simulink model "test_mdl_NI"  (R2018a)
settings: Solver=VariableStepAuto  StartTime=0.0  StopTime=10.0  RelTol=1e-3
(part 7 of 24)

== system test_mdl_NI/Subsystem/ABS_ESC/BrakeSysFeatures_2_Ox416 ==
  in_port : Inport
  Abs_B_Falt : Terminator
  BpedMove_D_Actl : Terminator
  BpedMove_No_Cnt : Terminator
  BrkBstrVac_B_Rq : Terminator
  BrkLamp_B_Rq : Terminator
  ChimeBrk_B_Rq : Terminator
  DrvAntiLckLamp_D_Rq : Terminator
  DrvHdcLampInfo_D_Rq : Terminator
  DrvHdcMsg_D_Rq : Terminator
  DrvHdcWarnInfo_D_Rq : Terminator
  DrvSlipCtlLamp_D_Rq : Terminator
  DrvSlipCtlMde_D_Ind : Terminator
  HILL_DESC_MC : Terminator
  HdcMde_D_Actl : Terminator
  HsaMde_D_Mem : Terminator
  RearDiffElckrOpen_B_Rq : Terminator
  RearDiffLck_Tq2_RqMx : Terminator
  StabCtlBrk_B_Avail : Terminator
  TCMode : Terminator
  TRLR_SWAY_CONFIG_STAT : Terminator
  TRLR_SWAY_EVNT_IN_PROG : Terminator
  bus_selector : BusSelector  OutputSignals=Abs_B_Falt,BpedMove_D_Actl,BpedMove_No_Cnt,BrkBstrVac_B_Rq,BrkLamp_B_Rq,ChimeBrk_B_Rq,DrvAntiLckLamp_D_Rq,DrvHdcLampInfo_D_Rq,DrvHdcMsg_D_Rq,DrvHdcWarnInfo_D_Rq,DrvSlipCtlLamp_D_Rq,DrvSlipCtlMde_D_Ind,HILL_DESC_MC,HdcMde_D_Actl,HsaMde_D_Mem,RearDiffElckrOpen_B_Rq,RearDiffLck_Tq2_RqMx,StabCtlBrk_B_Avail,TCMode,TRLR_SWAY_CONFIG_STAT,TRLR_SWAY_EVNT_IN_PROG
  wires:
  in_port/1 -> bus_selector/1  "BrakeSysFeatures_2_Ox416"
  bus_selector/1 -> Abs_B_Falt/1  "<Abs_B_Falt>"
  bus_selector/2 -> BpedMove_D_Actl/1  "<BpedMove_D_Actl>"
  bus_selector/3 -> BpedMove_No_Cnt/1  "<BpedMove_No_Cnt>"
  bus_selector/4 -> BrkBstrVac_B_Rq/1  "<BrkBstrVac_B_Rq>"
  bus_selector/5 -> BrkLamp_B_Rq/1  "<BrkLamp_B_Rq>"
  bus_selector/6 -> ChimeBrk_B_Rq/1  "<ChimeBrk_B_Rq>"
  bus_selector/7 -> DrvAntiLckLamp_D_Rq/1  "<DrvAntiLckLamp_D_Rq>"
  bus_selector/8 -> DrvHdcLampInfo_D_Rq/1  "<DrvHdcLampInfo_D_Rq>"
  bus_selector/9 -> DrvHdcMsg_D_Rq/1  "<DrvHdcMsg_D_Rq>"
  bus_selector/10 -> DrvHdcWarnInfo_D_Rq/1  "<DrvHdcWarnInfo_D_Rq>"
  bus_selector/11 -> DrvSlipCtlLamp_D_Rq/1  "<DrvSlipCtlLamp_D_Rq>"
  bus_selector/12 -> DrvSlipCtlMde_D_Ind/1  "<DrvSlipCtlMde_D_Ind>"
  bus_selector/13 -> HILL_DESC_MC/1  "<HILL_DESC_MC>"
  bus_selector/14 -> HdcMde_D_Actl/1  "<HdcMde_D_Actl>"
  bus_selector/15 -> HsaMde_D_Mem/1  "<HsaMde_D_Mem>"
  bus_selector/16 -> RearDiffElckrOpen_B_Rq/1  "<RearDiffElckrOpen_B_Rq>"
  bus_selector/17 -> RearDiffLck_Tq2_RqMx/1  "<RearDiffLck_Tq2_RqMx>"
  bus_selector/18 -> StabCtlBrk_B_Avail/1  "<StabCtlBrk_B_Avail>"
  bus_selector/19 -> TCMode/1  "<TCMode>"
  bus_selector/20 -> TRLR_SWAY_CONFIG_STAT/1  "<TRLR_SWAY_CONFIG_STAT>"
  bus_selector/21 -> TRLR_SWAY_EVNT_IN_PROG/1  "<TRLR_SWAY_EVNT_IN_PROG>"

== system test_mdl_NI/Subsystem/ABS_ESC/BrakeSysFeatures_3_Ox41E ==
  in_port : Inport
  AirDamUp_B_RqBrk : Terminator
  ApaBrk_D_Stat : Terminator
  AutoHoldMde_D_Ind : Terminator
  AutoHoldMsgTxt_D_Rq : Terminator
  AutoHoldSwMde_B_Ind : Terminator
  BrkBstrVac_D_Stat : Terminator
  CtaBrk_D_Stat : Terminator
  DrvSlipCtlMdeMsg_D_Rq : Terminator
  DrvSlipCtlOffLamp_D_Rq : Terminator
  RbaBrk_D_Stat : Terminator
  SelDrvMdeAwd_D_Rq : Terminator
  SelDrvMdeChassis2_D_Rq : Terminator
  SelDrvMdeChassis_D_Rq : Terminator
  TrailCtlMsgTxt_D_Rq : Terminator
  TrailCtl_D_Stat : Terminator
  bus_selector : BusSelector  OutputSignals=AirDamUp_B_RqBrk,ApaBrk_D_Stat,AutoHoldMde_D_Ind,AutoHoldMsgTxt_D_Rq,AutoHoldSwMde_B_Ind,BrkBstrVac_D_Stat,CtaBrk_D_Stat,DrvSlipCtlMdeMsg_D_Rq,DrvSlipCtlOffLamp_D_Rq,RbaBrk_D_Stat,SelDrvMdeAwd_D_Rq,SelDrvMdeChassis2_D_Rq,SelDrvMdeChassis_D_Rq,TrailCtlMsgTxt_D_Rq,TrailCtl_D_Stat
  wires:
  in_port/1 -> bus_selector/1  "BrakeSysFeatures_3_Ox41E"
  bus_selector/1 -> AirDamUp_B_RqBrk/1  "<AirDamUp_B_RqBrk>"
  bus_selector/2 -> ApaBrk_D_Stat/1  "<ApaBrk_D_Stat>"
  bus_selector/3 -> AutoHoldMde_D_Ind/1  "<AutoHoldMde_D_Ind>"
  bus_selector/4 -> AutoHoldMsgTxt_D_Rq/1  "<AutoHoldMsgTxt_D_Rq>"
  bus_selector/5 -> AutoHoldSwMde_B_Ind/1  "<AutoHoldSwMde_B_Ind>"
  bus_selector/6 -> BrkBstrVac_D_Stat/1  "<BrkBstrVac_D_Stat>"
  bus_selector/7 -> CtaBrk_D_Stat/1  "<CtaBrk_D_Stat>"
  bus_selector/8 -> DrvSlipCtlMdeMsg_D_Rq/1  "<DrvSlipCtlMdeMsg_D_Rq>"
  bus_selector/9 -> DrvSlipCtlOffLamp_D_Rq/1  "<DrvSlipCtlOffLamp_D_Rq>"
  bus_selector/10 -> RbaBrk_D_Stat/1  "<RbaBrk_D_Stat>"
  bus_selector/11 -> SelDrvMdeAwd_D_Rq/1  "<SelDrvMdeAwd_D_Rq>"
  bus_selector/12 -> SelDrvMdeChassis2_D_Rq/1  "<SelDrvMdeChassis2_D_Rq>"
  bus_selector/13 -> SelDrvMdeChassis_D_Rq/1  "<SelDrvMdeChassis_D_Rq>"
  bus_selector/14 -> TrailCtlMsgTxt_D_Rq/1  "<TrailCtlMsgTxt_D_Rq>"
  bus_selector/15 -> TrailCtl_D_Stat/1  "<TrailCtl_D_Stat>"

== system test_mdl_NI/Subsystem/ABS_ESC/BrakeSysFeatures_Ox415 ==
  in_port : Inport
  BrkFluidLvl_D_Stat : Terminator
  LsmcBrkDecel_D_Stat : Terminator
  VehStab_D_Stat : Terminator
  VehVActlBrk_D_Qf : Terminator
  VehVActlBrk_No_Cnt : Terminator
  VehVActlBrk_No_Cs : Terminator
  VehYawLin_W_Rq : Terminator
  VehYawNonLin_W_Rq : Terminator
  Veh_V_ActlBrk : Terminator
  bus_selector : BusSelector  OutputSignals=BrkFluidLvl_D_Stat,LsmcBrkDecel_D_Stat,VehStab_D_Stat,VehVActlBrk_D_Qf,VehVActlBrk_No_Cnt,VehVActlBrk_No_Cs,VehYawLin_W_Rq,VehYawNonLin_W_Rq,Veh_V_ActlBrk
  wires:
  in_port/1 -> bus_selector/1  "BrakeSysFeatures_Ox415"
  bus_selector/1 -> BrkFluidLvl_D_Stat/1  "<BrkFluidLvl_D_Stat>"
  bus_selector/2 -> LsmcBrkDecel_D_Stat/1  "<LsmcBrkDecel_D_Stat>"
  bus_selector/3 -> VehStab_D_Stat/1  "<VehStab_D_Stat>"
  bus_selector/4 -> VehVActlBrk_D_Qf/1  "<VehVActlBrk_D_Qf>"
  bus_selector/5 -> VehVActlBrk_No_Cnt/1  "<VehVActlBrk_No_Cnt>"
  bus_selector/6 -> VehVActlBrk_No_Cs/1  "<VehVActlBrk_No_Cs>"
  bus_selector/7 -> VehYawLin_W_Rq/1  "<VehYawLin_W_Rq>"
  bus_selector/8 -> VehYawNonLin_W_Rq/1  "<VehYawNonLin_W_Rq>"
  bus_selector/9 -> Veh_V_ActlBrk/1  "<Veh_V_ActlBrk>"

== system test_mdl_NI/Subsystem/ABS_ESC/DesiredTorqBrk_2_Ox214 ==
  in_port : Inport
  PrplWhlTot_Tq_RqMn : Terminator
  PrplWhlTqRqMn_No_Cnt : Terminator
  PrplWhlTqRqMn_No_Cs : Terminator
  RgenBrkDynoMde_B_Actl : Terminator
  RgenTqFalt_B_Actl : Terminator
  bus_selector : BusSelector  OutputSignals=PrplWhlTot_Tq_RqMn,PrplWhlTqRqMn_No_Cnt,PrplWhlTqRqMn_No_Cs,RgenBrkDynoMde_B_Actl,RgenTqFalt_B_Actl
  wires:
  in_port/1 -> bus_selector/1  "DesiredTorqBrk_2_Ox214"
  bus_selector/1 -> PrplWhlTot_Tq_RqMn/1  "<PrplWhlTot_Tq_RqMn>"
  bus_selector/2 -> PrplWhlTqRqMn_No_Cnt/1  "<PrplWhlTqRqMn_No_Cnt>"
  bus_selector/3 -> PrplWhlTqRqMn_No_Cs/1  "<PrplWhlTqRqMn_No_Cs>"
  bus_selector/4 -> RgenBrkDynoMde_B_Actl/1  "<RgenBrkDynoMde_B_Actl>"
  bus_selector/5 -> RgenTqFalt_B_Actl/1  "<RgenTqFalt_B_Actl>"

== system test_mdl_NI/Subsystem/ABS_ESC/DesiredTorqBrk_Ox213 ==
  in_port : Inport
  AbsActv_B_Actl : Terminator
  AccBrkActv_B_Actl : Terminator
  AccBrkDeny_B_Actl : Terminator
  AccBrkDis_B_Actl : Terminator
  AccBrkPrchgActv_B_Actl : Terminator
  AccBrkTotTqMn_B_Actl : Terminator
  AccBrkWarm_B_Actl : Terminator
  AccDis_B_ActlEpb : Terminator
  AccStopActv_B_ActlBrk : Terminator
  CcDis_B_Cmd : Terminator
  CmbbBaSensInc_B_Actl : Terminator
  CmbbBrkDecel_B_Actl : Terminator
  CmbbBrkDis_B_Actl : Terminator
  CmbbBrkPrchg_B_Actl : Terminator
  CmbbDeny_B_ActlBrk : Terminator
  LscmbBrkPrchg_B_Actl : Terminator
  LscmbbBaSensInc_B_Actl : Terminator
  LscmbbBrkDecel_B_Actl : Terminator
  LscmbbBrkDis_B_Actl : Terminator
  LscmbbDeny_B_ActlBrk : Terminator
  LscmbbMntr_B_Err : Terminator
  PrkBrkMsgTxt_D_Rq : Terminator
  PrkBrkRedLamp_D_Rq : Terminator
  PrkBrkStatus : Terminator
  PrkBrkYwLamp_D_Rq : Terminator
  PrplDrgCtlActv_B_Actl : Terminator
  PrplWhlTot_Tq_RqMx : Terminator
  StabCtlBrkActv_B_Actl : Terminator
  TracCtlPtActv_B_Actl : Terminator
  VehLongOvrGnd_A_Est : Terminator
  VehStop_D_Stat : Terminator
  bus_selector : BusSelector  OutputSignals=AbsActv_B_Actl,AccBrkActv_B_Actl,AccBrkDeny_B_Actl,AccBrkDis_B_Actl,AccBrkPrchgActv_B_Actl,AccBrkTotTqMn_B_Actl,AccBrkWarm_B_Actl,AccDis_B_ActlEpb,AccStopActv_B_ActlBrk,CcDis_B_Cmd,CmbbBaSensInc_B_Actl,CmbbBrkDecel_B_Actl,CmbbBrkDis_B_Actl,CmbbBrkPrchg_B_Actl,CmbbDeny_B_ActlBrk,LscmbBrkPrchg_B_Actl,LscmbbBaSensInc_B_Actl,LscmbbBrkDecel_B_Actl,LscmbbBrkDis_B_Actl,LscmbbDeny_B_ActlBrk,LscmbbMntr_B_Err,PrkBrkMsgTxt_D_Rq,PrkBrkRedLamp_D_Rq,PrkBrkStatus,PrkBrkYwLamp_D_Rq,PrplDrgCtlActv_B_Actl,PrplWhlTot_Tq_RqMx,StabCtlBrkActv_B_Actl,TracCtlPtActv_B_Actl,VehLongOvrGnd_A_Est,VehStop_D_Stat
  wires:
  in_port/1 -> bus_selector/1  "DesiredTorqBrk_Ox213"
  bus_selector/1 -> AbsActv_B_Actl/1  "<AbsActv_B_Actl>"
  bus_selector/2 -> AccBrkActv_B_Actl/1  "<AccBrkActv_B_Actl>"
  bus_selector/3 -> AccBrkDeny_B_Actl/1  "<AccBrkDeny_B_Actl>"
  bus_selector/4 -> AccBrkDis_B_Actl/1  "<AccBrkDis_B_Actl>"
  bus_selector/5 -> AccBrkPrchgActv_B_Actl/1  "<AccBrkPrchgActv_B_Actl>"
  bus_selector/6 -> AccBrkTotTqMn_B_Actl/1  "<AccBrkTotTqMn_B_Actl>"
  bus_selector/7 -> AccBrkWarm_B_Actl/1  "<AccBrkWarm_B_Actl>"
  bus_selector/8 -> AccDis_B_ActlEpb/1  "<AccDis_B_ActlEpb>"
  bus_selector/9 -> AccStopActv_B_ActlBrk/1  "<AccStopActv_B_ActlBrk>"
  bus_selector/10 -> CcDis_B_Cmd/1  "<CcDis_B_Cmd>"
  bus_selector/11 -> CmbbBaSensInc_B_Actl/1  "<CmbbBaSensInc_B_Actl>"
  bus_selector/12 -> CmbbBrkDecel_B_Actl/1  "<CmbbBrkDecel_B_Actl>"
  bus_selector/13 -> CmbbBrkDis_B_Actl/1  "<CmbbBrkDis_B_Actl>"
  bus_selector/14 -> CmbbBrkPrchg_B_Actl/1  "<CmbbBrkPrchg_B_Actl>"
  bus_selector/15 -> CmbbDeny_B_ActlBrk/1  "<CmbbDeny_B_ActlBrk>"
  bus_selector/16 -> LscmbBrkPrchg_B_Actl/1  "<LscmbBrkPrchg_B_Actl>"
  bus_selector/17 -> LscmbbBaSensInc_B_Actl/1  "<LscmbbBaSensInc_B_Actl>"
  bus_selector/18 -> LscmbbBrkDecel_B_Actl/1  "<LscmbbBrkDecel_B_Actl>"
  bus_selector/19 -> LscmbbBrkDis_B_Actl/1  "<LscmbbBrkDis_B_Actl>"
  bus_selector/20 -> LscmbbDeny_B_ActlBrk/1  "<LscmbbDeny_B_ActlBrk>"
  bus_selector/21 -> LscmbbMntr_B_Err/1  "<LscmbbMntr_B_Err>"
  bus_selector/22 -> PrkBrkMsgTxt_D_Rq/1  "<PrkBrkMsgTxt_D_Rq>"
  bus_selector/23 -> PrkBrkRedLamp_D_Rq/1  "<PrkBrkRedLamp_D_Rq>"
  bus_selector/24 -> PrkBrkStatus/1  "<PrkBrkStatus>"
  bus_selector/25 -> PrkBrkYwLamp_D_Rq/1  "<PrkBrkYwLamp_D_Rq>"
  bus_selector/26 -> PrplDrgCtlActv_B_Actl/1  "<PrplDrgCtlActv_B_Actl>"
  bus_selector/27 -> PrplWhlTot_Tq_RqMx/1  "<PrplWhlTot_Tq_RqMx>"
  bus_selector/28 -> StabCtlBrkActv_B_Actl/1  "<StabCtlBrkActv_B_Actl>"
  bus_selector/29 -> TracCtlPtActv_B_Actl/1  "<TracCtlPtActv_B_Actl>"
  bus_selector/30 -> VehLongOvrGnd_A_Est/1  "<VehLongOvrGnd_A_Est>"
  bus_selector/31 -> VehStop_D_Stat/1  "<VehStop_D_Stat>"

== system test_mdl_NI/Subsystem/ABS_ESC/Global_PATS_SubTarget_Ox49 ==
  in_port : Inport
  bus_selector : BusSelector  OutputSignals=immoSubTarget1Cmd_T1,immoSubTarget1Data_T1
  immoSubTarget1Cmd_T1 : Terminator
  immoSubTarget1Data_T1 : Terminator
  wires:
  in_port/1 -> bus_selector/1  "Global_PATS_SubTarget_Ox49"
  bus_selector/1 -> immoSubTarget1Cmd_T1/1  "<immoSubTarget1Cmd_T1>"
  bus_selector/2 -> immoSubTarget1Data_T1/1  "<immoSubTarget1Data_T1>"

== system test_mdl_NI/Subsystem/ABS_ESC/OTAPhysABStoGWM_ECG_Ox1B936028 ==
  in_port : Inport
  OTAPhysABStoGWM_ECG : Terminator
  bus_selector : BusSelector  OutputSignals=OTAPhysABStoGWM_ECG
  wires:
  in_port/1 -> bus_selector/1  "OTAPhysABStoGWM_ECG_Ox1B936028"
  bus_selector/1 -> OTAPhysABStoGWM_ECG/1  "<OTAPhysABStoGWM_ECG>"

== system test_mdl_NI/Subsystem/ABS_ESC/PARSEDPhysABStoGWM_ECG_Ox1BA36028 ==
  in_port : Inport
  PARSEDPhysABStoGWM_ECG : Terminator
  bus_selector : BusSelector  OutputSignals=PARSEDPhysABStoGWM_ECG
  wires:
  in_port/1 -> bus_selector/1  "PARSEDPhysABStoGWM_ECG_Ox1BA36028"
  bus_selector/1 -> PARSEDPhysABStoGWM_ECG/1  "<PARSEDPhysABStoGWM_ECG>"

== system test_mdl_NI/Subsystem/ABS_ESC/PARSEDPushABStoGWM_ECG_Ox1BB36028 ==
  in_port : Inport
  PARSEDPhysABS2toGWM_ECG : Terminator
  bus_selector : BusSelector  OutputSignals=PARSEDPhysABS2toGWM_ECG
  wires:
  in_port/1 -> bus_selector/1  "PARSEDPushABStoGWM_ECG_Ox1BB36028"
  bus_selector/1 -> PARSEDPhysABS2toGWM_ECG/1  "<PARSEDPhysABS2toGWM_ECG>"

== system test_mdl_NI/Subsystem/ABS_ESC/SelectDriveModeData2_Ox44E ==
  in_port : Inport
  SelDrvMdePos01_D_Stat : Terminator
  SelDrvMdePos02_D_Stat : Terminator
  SelDrvMdePos03_D_Stat : Terminator
  SelDrvMdePos04_D_Stat : Terminator
  SelDrvMdePos05_D_Stat : Terminator
  SelDrvMdePos06_D_Stat : Terminator
  SelDrvMdePos07_D_Stat : Terminator
  SelDrvMdePos08_D_Stat : Terminator
  SelDrvMdePos09_D_Stat : Terminator
  SelDrvMdePos10_D_Stat : Terminator
  SelDrvMdePos11_D_Stat : Terminator
  SelDrvMdePos12_D_Stat : Terminator
  bus_selector : BusSelector  OutputSignals=SelDrvMdePos01_D_Stat,SelDrvMdePos02_D_Stat,SelDrvMdePos03_D_Stat,SelDrvMdePos04_D_Stat,SelDrvMdePos05_D_Stat,SelDrvMdePos06_D_Stat,SelDrvMdePos07_D_Stat,SelDrvMdePos08_D_Stat,SelDrvMdePos09_D_Stat,SelDrvMdePos10_D_Stat,SelDrvMdePos11_D_Stat,SelDrvMdePos12_D_Stat
  wires:
  in_port/1 -> bus_selector/1  "SelectDriveModeData2_Ox44E"
  bus_selector/1 -> SelDrvMdePos01_D_Stat/1  "<SelDrvMdePos01_D_Stat>"
  bus_selector/2 -> SelDrvMdePos02_D_Stat/1  "<SelDrvMdePos02_D_Stat>"
  bus_selector/3 -> SelDrvMdePos03_D_Stat/1  "<SelDrvMdePos03_D_Stat>"
  bus_selector/4 -> SelDrvMdePos04_D_Stat/1  "<SelDrvMdePos04_D_Stat>"
  bus_selector/5 -> SelDrvMdePos05_D_Stat/1  "<SelDrvMdePos05_D_Stat>"
  bus_selector/6 -> SelDrvMdePos06_D_Stat/1  "<SelDrvMdePos06_D_Stat>"
  bus_selector/7 -> SelDrvMdePos07_D_Stat/1  "<SelDrvMdePos07_D_Stat>"
  bus_selector/8 -> SelDrvMdePos08_D_Stat/1  "<SelDrvMdePos08_D_Stat>"
  bus_selector/9 -> SelDrvMdePos09_D_Stat/1  "<SelDrvMdePos09_D_Stat>"
  bus_selector/10 -> SelDrvMdePos10_D_Stat/1  "<SelDrvMdePos10_D_Stat>"
  bus_selector/11 -> SelDrvMdePos11_D_Stat/1  "<SelDrvMdePos11_D_Stat>"
  bus_selector/12 -> SelDrvMdePos12_D_Stat/1  "<SelDrvMdePos12_D_Stat>"

== system test_mdl_NI/Subsystem/ABS_ESC/SelectDriveModeData_Ox420 ==
  in_port : Inport
  ActvDrvMde_D2_Stat : Terminator
  AutoEpbButtnOn_B_Stat : Terminator
  AutoEpbDsply_D_Stat : Terminator
  AutoEpbMsgTxt_D_Rq : Terminator
  AwdMde_D_RqBrk : Terminator
  SelDrvMdeMsgTxt_D_Rq : Terminator
  SelDrvMdePos01_B_Avail : Terminator
  SelDrvMdePos02_B_Avail : Terminator
  SelDrvMdePos03_B_Avail : Terminator
  SelDrvMdePos04_B_Avail : Terminator
  SelDrvMdePos05_B_Avail : Terminator
  SelDrvMdePos06_B_Avail : Terminator
  SelDrvMdePos07_B_Avail : Terminator
  SelDrvMdePos08_B_Avail : Terminator
  SelDrvMdePos09_B_Avail : Terminator
  SelDrvMdePos10_B_Avail : Terminator
  SelDrvMdePos11_B_Avail : Terminator
  SelDrvMdePos12_B_Avail : Terminator
  SelDrvMdePt_D_Rq : Terminator
  SelDrvMde_D2_Rq : Terminator
  SelDrvMde_D_Stat : Terminator
  bus_selector : BusSelector  OutputSignals=ActvDrvMde_D2_Stat,AutoEpbButtnOn_B_Stat,AutoEpbDsply_D_Stat,AutoEpbMsgTxt_D_Rq,AwdMde_D_RqBrk,SelDrvMdeMsgTxt_D_Rq,SelDrvMdePos01_B_Avail,SelDrvMdePos02_B_Avail,SelDrvMdePos03_B_Avail,SelDrvMdePos04_B_Avail,SelDrvMdePos05_B_Avail,SelDrvMdePos06_B_Avail,SelDrvMdePos07_B_Avail,SelDrvMdePos08_B_Avail,SelDrvMdePos09_B_Avail,SelDrvMdePos10_B_Avail,SelDrvMdePos11_B_Avail,SelDrvMdePos12_B_Avail,SelDrvMdePt_D_Rq,SelDrvMde_D2_Rq,SelDrvMde_D_Stat
  wires:
  in_port/1 -> bus_selector/1  "SelectDriveModeData_Ox420"
  bus_selector/1 -> ActvDrvMde_D2_Stat/1  "<ActvDrvMde_D2_Stat>"
  bus_selector/2 -> AutoEpbButtnOn_B_Stat/1  "<AutoEpbButtnOn_B_Stat>"
  bus_selector/3 -> AutoEpbDsply_D_Stat/1  "<AutoEpbDsply_D_Stat>"
  bus_selector/4 -> AutoEpbMsgTxt_D_Rq/1  "<AutoEpbMsgTxt_D_Rq>"
  bus_selector/5 -> AwdMde_D_RqBrk/1  "<AwdMde_D_RqBrk>"
  bus_selector/6 -> SelDrvMdeMsgTxt_D_Rq/1  "<SelDrvMdeMsgTxt_D_Rq>"
  bus_selector/7 -> SelDrvMdePos01_B_Avail/1  "<SelDrvMdePos01_B_Avail>"
  bus_selector/8 -> SelDrvMdePos02_B_Avail/1  "<SelDrvMdePos02_B_Avail>"
  bus_selector/9 -> SelDrvMdePos03_B_Avail/1  "<SelDrvMdePos03_B_Avail>"
  bus_selector/10 -> SelDrvMdePos04_B_Avail/1  "<SelDrvMdePos04_B_Avail>"
  bus_selector/11 -> SelDrvMdePos05_B_Avail/1  "<SelDrvMdePos05_B_Avail>"
  bus_selector/12 -> SelDrvMdePos06_B_Avail/1  "<SelDrvMdePos06_B_Avail>"
  bus_selector/13 -> SelDrvMdePos07_B_Avail/1  "<SelDrvMdePos07_B_Avail>"
  bus_selector/14 -> SelDrvMdePos08_B_Avail/1  "<SelDrvMdePos08_B_Avail>"
  bus_selector/15 -> SelDrvMdePos09_B_Avail/1  "<SelDrvMdePos09_B_Avail>"
  bus_selector/16 -> SelDrvMdePos10_B_Avail/1  "<SelDrvMdePos10_B_Avail>"
  bus_selector/17 -> SelDrvMdePos11_B_Avail/1  "<SelDrvMdePos11_B_Avail>"
  bus_selector/18 -> SelDrvMdePos12_B_Avail/1  "<SelDrvMdePos12_B_Avail>"
  bus_selector/19 -> SelDrvMdePt_D_Rq/1  "<SelDrvMdePt_D_Rq>"
  bus_selector/20 -> SelDrvMde_D2_Rq/1  "<SelDrvMde_D2_Rq>"
  bus_selector/21 -> SelDrvMde_D_Stat/1  "<SelDrvMde_D_Stat>"

== system test_mdl_NI/Subsystem/ABS_ESC/TesterPhysicalResABS_Ox768 ==
  in_port : Inport
  TesterPhysicalResABS : Terminator
  bus_selector : BusSelector  OutputSignals=TesterPhysicalResABS
  wires:
  in_port/1 -> bus_selector/1  "TesterPhysicalResABS_Ox768"
  bus_selector/1 -> TesterPhysicalResABS/1  "<TesterPhysicalResABS>"

== system test_mdl_NI/Subsystem/ABS_ESC/TrailerBrakeData_Ox412 ==
  in_port : Inport
  TrlrBrk_Pc_Rq : Terminator
  VehPtch_An_Dsply : Terminator
  VehRol_An_Dsply : Terminator
  bus_selector : BusSelector  OutputSignals=TrlrBrk_Pc_Rq,VehPtch_An_Dsply,VehRol_An_Dsply
  wires:
  in_port/1 -> bus_selector/1  "TrailerBrakeData_Ox412"
  bus_selector/1 -> TrlrBrk_Pc_Rq/1  "<TrlrBrk_Pc_Rq>"
  bus_selector/2 -> VehPtch_An_Dsply/1  "<VehPtch_An_Dsply>"
  bus_selector/3 -> VehRol_An_Dsply/1  "<VehRol_An_Dsply>"

== system test_mdl_NI/Subsystem/ABS_ESC/WheelData_Ox216 ==
  in_port : Inport
  BrkObdData_No_Actl : Terminator
  BrkObdIndex_No_Actl : Terminator
  WhlDirFl_D_Actl : Terminator
  WhlDirFr_D_Actl : Terminator
  WhlDirRl_D_Actl : Terminator
  WhlDirRr_D_Actl : Terminator
  WhlRotatFl_No_Cnt : Terminator
  WhlRotatFr_No_Cnt : Terminator
  WhlRotatRl_No_Cnt : Terminator
  WhlRotatRr_No_Cnt : Terminator
  bus_selector : BusSelector  OutputSignals=BrkObdData_No_Actl,BrkObdIndex_No_Actl,WhlDirFl_D_Actl,WhlDirFr_D_Actl,WhlDirRl_D_Actl,WhlDirRr_D_Actl,WhlRotatFl_No_Cnt,WhlRotatFr_No_Cnt,WhlRotatRl_No_Cnt,WhlRotatRr_No_Cnt
  wires:
  in_port/1 -> bus_selector/1  "WheelData_Ox216"
  bus_selector/1 -> BrkObdData_No_Actl/1  "<BrkObdData_No_Actl>"
  bus_selector/2 -> BrkObdIndex_No_Actl/1  "<BrkObdIndex_No_Actl>"
  bus_selector/3 -> WhlDirFl_D_Actl/1  "<WhlDirFl_D_Actl>"
  bus_selector/4 -> WhlDirFr_D_Actl/1  "<WhlDirFr_D_Actl>"
  bus_selector/5 -> WhlDirRl_D_Actl/1  "<WhlDirRl_D_Actl>"
  bus_selector/6 -> WhlDirRr_D_Actl/1  "<WhlDirRr_D_Actl>"
  bus_selector/7 -> WhlRotatFl_No_Cnt/1  "<WhlRotatFl_No_Cnt>"
  bus_selector/8 -> WhlRotatFr_No_Cnt/1  "<WhlRotatFr_No_Cnt>"
  bus_selector/9 -> WhlRotatRl_No_Cnt/1  "<WhlRotatRl_No_Cnt>"
  bus_selector/10 -> WhlRotatRr_No_Cnt/1  "<WhlRotatRr_No_Cnt>"

== system test_mdl_NI/Subsystem/ABS_ESC/WheelSpeed_Ox217 ==
  in_port : Inport
  WhlFl_W_Meas : Terminator
  WhlFr_W_Meas : Terminator
  WhlRl_W_Meas : Terminator
  WhlRr_W_Meas : Terminator
  bus_selector : BusSelector  OutputSignals=WhlFl_W_Meas,WhlFr_W_Meas,WhlRl_W_Meas,WhlRr_W_Meas
  wires:
  in_port/1 -> bus_selector/1  "WheelSpeed_Ox217"
  bus_selector/1 -> WhlFl_W_Meas/1  "<WhlFl_W_Meas>"
  bus_selector/2 -> WhlFr_W_Meas/1  "<WhlFr_W_Meas>"
  bus_selector/3 -> WhlRl_W_Meas/1  "<WhlRl_W_Meas>"
  bus_selector/4 -> WhlRr_W_Meas/1  "<WhlRr_W_Meas>"

== system test_mdl_NI/Subsystem/CMR_DSMC/CMR_DSMC_AutoSar_NetwrkMgt_Ox5DF ==
  in_port : Inport
  CMR_DSMC_AutoSarNMControl : Terminator
  CMR_DSMC_AutoSarNMNodeId : Terminator
  CMR_DSMC_AutoSarNMReserve2 : Terminator
  CMR_DSMC_AutoSarNMReserve3 : Terminator
  CMR_DSMC_AutoSarNMReserve4 : Terminator
  CMR_DSMC_AutoSarNMReserved : Terminator
  CMR_DSMC_GWNMProxY : Terminator
  CMR_DSMC_GWOnBoardTester : Terminator
  bus_selector : BusSelector  OutputSignals=CMR_DSMC_AutoSarNMControl,CMR_DSMC_AutoSarNMNodeId,CMR_DSMC_AutoSarNMReserve2,CMR_DSMC_AutoSarNMReserve3,CMR_DSMC_AutoSarNMReserve4,CMR_DSMC_AutoSarNMReserved,CMR_DSMC_GWNMProxY,CMR_DSMC_GWOnBoardTester
  wires:
  in_port/1 -> bus_selector/1  "CMR_DSMC_AutoSar_NetwrkMgt_Ox5DF"
  bus_selector/1 -> CMR_DSMC_AutoSarNMControl/1  "<CMR_DSMC_AutoSarNMControl>"
  bus_selector/2 -> CMR_DSMC_AutoSarNMNodeId/1  "<CMR_DSMC_AutoSarNMNodeId>"
  bus_selector/3 -> CMR_DSMC_AutoSarNMReserve2/1  "<CMR_DSMC_AutoSarNMReserve2>"
  bus_selector/4 -> CMR_DSMC_AutoSarNMReserve3/1  "<CMR_DSMC_AutoSarNMReserve3>"
  bus_selector/5 -> CMR_DSMC_AutoSarNMReserve4/1  "<CMR_DSMC_AutoSarNMReserve4>"
  bus_selector/6 -> CMR_DSMC_AutoSarNMReserved/1  "<CMR_DSMC_AutoSarNMReserved>"
  bus_selector/7 -> CMR_DSMC_GWNMProxY/1  "<CMR_DSMC_GWNMProxY>"
  bus_selector/8 -> CMR_DSMC_GWOnBoardTester/1  "<CMR_DSMC_GWOnBoardTester>"

== system test_mdl_NI/Subsystem/CMR_DSMC/DrvStatMonData_Ox450 ==
  in_port : Inport
  DrvAlertSt_D_Stat : Terminator
  DrvAttentZone_D_Stat : Terminator
  DrvCamDrvIR_D_Stat : Terminator
  DrvCamPassIR_D_Stat : Terminator
  DrvCamera_D_Stat : Terminator
  DrvEngLvlConfid_D_Stat : Terminator
  DrvEngageLevel_D_Stat : Terminator
  DrvEngageLevel_No_Cnt : Terminator
  DrvEngageLevel_No_Cs : Terminator
  DrvImpLvlConfid_D_Stat : Terminator
  DrvImpairLvl_D_Stat : Terminator
  bus_selector : BusSelector  OutputSignals=DrvAlertSt_D_Stat,DrvAttentZone_D_Stat,DrvCamDrvIR_D_Stat,DrvCamPassIR_D_Stat,DrvCamera_D_Stat,DrvEngLvlConfid_D_Stat,DrvEngageLevel_D_Stat,DrvEngageLevel_No_Cnt,DrvEngageLevel_No_Cs,DrvImpLvlConfid_D_Stat,DrvImpairLvl_D_Stat
  wires:
  in_port/1 -> bus_selector/1  "DrvStatMonData_Ox450"
  bus_selector/1 -> DrvAlertSt_D_Stat/1  "<DrvAlertSt_D_Stat>"
  bus_selector/2 -> DrvAttentZone_D_Stat/1  "<DrvAttentZone_D_Stat>"
  bus_selector/3 -> DrvCamDrvIR_D_Stat/1  "<DrvCamDrvIR_D_Stat>"
  bus_selector/4 -> DrvCamPassIR_D_Stat/1  "<DrvCamPassIR_D_Stat>"
  bus_selector/5 -> DrvCamera_D_Stat/1  "<DrvCamera_D_Stat>"
  bus_selector/6 -> DrvEngLvlConfid_D_Stat/1  "<DrvEngLvlConfid_D_Stat>"
  bus_selector/7 -> DrvEngageLevel_D_Stat/1  "<DrvEngageLevel_D_Stat>"
  bus_selector/8 -> DrvEngageLevel_No_Cnt/1  "<DrvEngageLevel_No_Cnt>"
  bus_selector/9 -> DrvEngageLevel_No_Cs/1  "<DrvEngageLevel_No_Cs>"
  bus_selector/10 -> DrvImpLvlConfid_D_Stat/1  "<DrvImpLvlConfid_D_Stat>"
  bus_selector/11 -> DrvImpairLvl_D_Stat/1  "<DrvImpairLvl_D_Stat>"

== system test_mdl_NI/Subsystem/CMR_DSMC/TesterPhysicalResCMR_DSMC_Ox7C9 ==
  in_port : Inport
  TesterPhysicalResCMR_DSMC : Terminator
  bus_selector : BusSelector  OutputSignals=TesterPhysicalResCMR_DSMC
  wires:
  in_port/1 -> bus_selector/1  "TesterPhysicalResCMR_DSMC_Ox7C9"
  bus_selector/1 -> TesterPhysicalResCMR_DSMC/1  "<TesterPhysicalResCMR_DSMC>"

== system test_mdl_NI/Subsystem/ECM_Diesel/CGEA_Urea_Strategy_Ox14C ==
  in_port : Inport
  DieslPrtcWarn_D_Rq : Terminator
  UreaLvlQlty_D_RqDsply : Terminator
  UreaLvlTxtWarn_D_Rq : Terminator
  UreaLvlTxt_D_RqDsply : Terminator
  UreaLvl_Pc_Actl : Terminator
  UreaQltyFlg_B_RqDsply : Terminator
  UreaQltySysWarn_D_Rq : Terminator
  UreaQltySys_D_RqDsply : Terminator
  VehUreaRnge2_L_DsplyMx : Terminator
  VehUreaWarn_V_DsplyMx : Terminator
  bus_selector : BusSelector  OutputSignals=DieslPrtcWarn_D_Rq,UreaLvlQlty_D_RqDsply,UreaLvlTxtWarn_D_Rq,UreaLvlTxt_D_RqDsply,UreaLvl_Pc_Actl,UreaQltyFlg_B_RqDsply,UreaQltySysWarn_D_Rq,UreaQltySys_D_RqDsply,VehUreaRnge2_L_DsplyMx,VehUreaWarn_V_DsplyMx
  wires:
  in_port/1 -> bus_selector/1  "CGEA_Urea_Strategy_Ox14C"
  bus_selector/1 -> DieslPrtcWarn_D_Rq/1  "<DieslPrtcWarn_D_Rq>"
  bus_selector/2 -> UreaLvlQlty_D_RqDsply/1  "<UreaLvlQlty_D_RqDsply>"
  bus_selector/3 -> UreaLvlTxtWarn_D_Rq/1  "<UreaLvlTxtWarn_D_Rq>"
  bus_selector/4 -> UreaLvlTxt_D_RqDsply/1  "<UreaLvlTxt_D_RqDsply>"
  bus_selector/5 -> UreaLvl_Pc_Actl/1  "<UreaLvl_Pc_Actl>"
  bus_selector/6 -> UreaQltyFlg_B_RqDsply/1  "<UreaQltyFlg_B_RqDsply>"
  bus_selector/7 -> UreaQltySysWarn_D_Rq/1  "<UreaQltySysWarn_D_Rq>"
  bus_selector/8 -> UreaQltySys_D_RqDsply/1  "<UreaQltySys_D_RqDsply>"
  bus_selector/9 -> VehUreaRnge2_L_DsplyMx/1  "<VehUreaRnge2_L_DsplyMx>"
  bus_selector/10 -> VehUreaWarn_V_DsplyMx/1  "<VehUreaWarn_V_DsplyMx>"

== system test_mdl_NI/Subsystem/ECM_Diesel/EffDrvModeData_Ox44A ==
  in_port : Inport
  EdmCmplnc_B_Dsply : Terminator
  EdmCmplnc_Pc_Dsply : Terminator
  EdmCurrent_Fe_Dsply : Terminator
  EdmLamp_D_Dsply : Terminator
  EdmMsgTxt_D_Rq : Terminator
  EdmPrev_Fe_Dsply : Terminator
  EdmSailMdeOn_B_Stat : Terminator
  EdmVeh_V_Dsply : Terminator
  bus_selector : BusSelector  OutputSignals=EdmCmplnc_B_Dsply,EdmCmplnc_Pc_Dsply,EdmCurrent_Fe_Dsply,EdmLamp_D_Dsply,EdmMsgTxt_D_Rq,EdmPrev_Fe_Dsply,EdmSailMdeOn_B_Stat,EdmVeh_V_Dsply
  wires:
  in_port/1 -> bus_selector/1  "EffDrvModeData_Ox44A"
  bus_selector/1 -> EdmCmplnc_B_Dsply/1  "<EdmCmplnc_B_Dsply>"
  bus_selector/2 -> EdmCmplnc_Pc_Dsply/1  "<EdmCmplnc_Pc_Dsply>"
  bus_selector/3 -> EdmCurrent_Fe_Dsply/1  "<EdmCurrent_Fe_Dsply>"
  bus_selector/4 -> EdmLamp_D_Dsply/1  "<EdmLamp_D_Dsply>"
  bus_selector/5 -> EdmMsgTxt_D_Rq/1  "<EdmMsgTxt_D_Rq>"
  bus_selector/6 -> EdmPrev_Fe_Dsply/1  "<EdmPrev_Fe_Dsply>"
  bus_selector/7 -> EdmSailMdeOn_B_Stat/1  "<EdmSailMdeOn_B_Stat>"
  bus_selector/8 -> EdmVeh_V_Dsply/1  "<EdmVeh_V_Dsply>"

== system test_mdl_NI/Subsystem/ECM_Diesel/EngBrakeData_Ox165 ==
  in_port : Inport
  AccEngStat_D_Actl : Terminator
  AccStopMde_D_Rq : Terminator
  BPedDrvAppl_D_QF : Terminator
  BpedDrvAppl_D_Actl : Terminator
  CcMde_D_Actl : Terminator
  CcOvrrdActv_B_Actl : Terminator
  CcStat_D_Actl : Terminator
  CmbbDeny_B_ActlPrpl : Terminator
  CmbbEngTqMn_B_Actl : Terminator
  EngAout_N_MnAllw : Terminator
  PrplTqMnSat_B_Actl : Terminator
  Veh_V_DsplyCcSet : Terminator
  bus_selector : BusSelector  OutputSignals=AccEngStat_D_Actl,AccStopMde_D_Rq,BPedDrvAppl_D_QF,BpedDrvAppl_D_Actl,CcMde_D_Actl,CcOvrrdActv_B_Actl,CcStat_D_Actl,CmbbDeny_B_ActlPrpl,CmbbEngTqMn_B_Actl,EngAout_N_MnAllw,PrplTqMnSat_B_Actl,Veh_V_DsplyCcSet
  wires:
  in_port/1 -> bus_selector/1  "EngBrakeData_Ox165"
  bus_selector/1 -> AccEngStat_D_Actl/1  "<AccEngStat_D_Actl>"
  bus_selector/2 -> AccStopMde_D_Rq/1  "<AccStopMde_D_Rq>"
  bus_selector/3 -> BPedDrvAppl_D_QF/1  "<BPedDrvAppl_D_QF>"
  bus_selector/4 -> BpedDrvAppl_D_Actl/1  "<BpedDrvAppl_D_Actl>"
  bus_selector/5 -> CcMde_D_Actl/1  "<CcMde_D_Actl>"
  bus_selector/6 -> CcOvrrdActv_B_Actl/1  "<CcOvrrdActv_B_Actl>"
  bus_selector/7 -> CcStat_D_Actl/1  "<CcStat_D_Actl>"
  bus_selector/8 -> CmbbDeny_B_ActlPrpl/1  "<CmbbDeny_B_ActlPrpl>"
  bus_selector/9 -> CmbbEngTqMn_B_Actl/1  "<CmbbEngTqMn_B_Actl>"
  bus_selector/10 -> EngAout_N_MnAllw/1  "<EngAout_N_MnAllw>"
  bus_selector/11 -> PrplTqMnSat_B_Actl/1  "<PrplTqMnSat_B_Actl>"
  bus_selector/12 -> Veh_V_DsplyCcSet/1  "<Veh_V_DsplyCcSet>"

== system test_mdl_NI/Subsystem/ECM_Diesel/EngVehicleSpThrottle2_Ox202 ==
  in_port : Inport
  GearRvrse_D_Actl : Terminator
  StrtrMtrCtlMsgTxt_D2_Rq : Terminator
  StrtrMtrCtlMsgTxt_D_Rq : Terminator
  StrtrMtrDlyStrt_B_Stat : Terminator
  VehVActlEng_D_Qf : Terminator
  VehVActlEng_No_Cnt : Terminator
  VehVActlEng_No_Cs : Terminator
  VehVTrlrAid_B_Avail : Terminator
  Veh_V_ActlEng : Terminator
  Veh_V_RqCcSet : Terminator
  bus_selector : BusSelector  OutputSignals=GearRvrse_D_Actl,StrtrMtrCtlMsgTxt_D2_Rq,StrtrMtrCtlMsgTxt_D_Rq,StrtrMtrDlyStrt_B_Stat,VehVActlEng_D_Qf,VehVActlEng_No_Cnt,VehVActlEng_No_Cs,VehVTrlrAid_B_Avail,Veh_V_ActlEng,Veh_V_RqCcSet
  wires:
  in_port/1 -> bus_selector/1  "EngVehicleSpThrottle2_Ox202"
  bus_selector/1 -> GearRvrse_D_Actl/1  "<GearRvrse_D_Actl>"
  bus_selector/2 -> StrtrMtrCtlMsgTxt_D2_Rq/1  "<StrtrMtrCtlMsgTxt_D2_Rq>"
  bus_selector/3 -> StrtrMtrCtlMsgTxt_D_Rq/1  "<StrtrMtrCtlMsgTxt_D_Rq>"
  bus_selector/4 -> StrtrMtrDlyStrt_B_Stat/1  "<StrtrMtrDlyStrt_B_Stat>"
  bus_selector/5 -> VehVActlEng_D_Qf/1  "<VehVActlEng_D_Qf>"
  bus_selector/6 -> VehVActlEng_No_Cnt/1  "<VehVActlEng_No_Cnt>"
  bus_selector/7 -> VehVActlEng_No_Cs/1  "<VehVActlEng_No_Cs>"
  bus_selector/8 -> VehVTrlrAid_B_Avail/1  "<VehVTrlrAid_B_Avail>"
  bus_selector/9 -> Veh_V_ActlEng/1  "<Veh_V_ActlEng>"
  bus_selector/10 -> Veh_V_RqCcSet/1  "<Veh_V_RqCcSet>"

== system test_mdl_NI/Subsystem/ECM_Diesel/EngVehicleSpThrottle_Ox204 ==
  in_port : Inport
  ApedPosPcActl_D_Qf : Terminator
  ApedPosPcActl_No_Cnt : Terminator
  ApedPosPcActl_No_Cs : Terminator
  ApedPos_PcRate_ActlArb : Terminator
  ApedPos_Pc_ActlArb : Terminator
  EngAout3_N_Actl : Terminator
  EngAoutNActl_D_QF : Terminator
  EngAout_N_Actl : Terminator
  bus_selector : BusSelector  OutputSignals=ApedPosPcActl_D_Qf,ApedPosPcActl_No_Cnt,ApedPosPcActl_No_Cs,ApedPos_PcRate_ActlArb,ApedPos_Pc_ActlArb,EngAout3_N_Actl,EngAoutNActl_D_QF,EngAout_N_Actl
  wires:
  in_port/1 -> bus_selector/1  "EngVehicleSpThrottle_Ox204"
  bus_selector/1 -> ApedPosPcActl_D_Qf/1  "<ApedPosPcActl_D_Qf>"
  bus_selector/2 -> ApedPosPcActl_No_Cnt/1  "<ApedPosPcActl_No_Cnt>"
  bus_selector/3 -> ApedPosPcActl_No_Cs/1  "<ApedPosPcActl_No_Cs>"
  bus_selector/4 -> ApedPos_PcRate_ActlArb/1  "<ApedPos_PcRate_ActlArb>"
  bus_selector/5 -> ApedPos_Pc_ActlArb/1  "<ApedPos_Pc_ActlArb>"
  bus_selector/6 -> EngAout3_N_Actl/1  "<EngAout3_N_Actl>"
  bus_selector/7 -> EngAoutNActl_D_QF/1  "<EngAoutNActl_D_QF>"
  bus_selector/8 -> EngAout_N_Actl/1  "<EngAout_N_Actl>"

== system test_mdl_NI/Subsystem/ECM_Diesel/EngineClimateData_Ox178 ==
  in_port : Inport
  AirAmbTe_D_Qf : Terminator
  AirAmb_P_Actl : Terminator
  AirAmb_Te_Actl : Terminator
  AirAmb_Te_ActlFilt : Terminator
  AslChime_B_Rq : Terminator
  AslIconDsply_D_Rq : Terminator
  DynoMde_B_Cmd : Terminator
  EcssLamp_D_RqDsply : Terminator
  EngAout_Aa_Actl : Terminator
  GasPrtc_D_RqDsply : Terminator
  HvacHtrCore2_Te_Actl : Terminator
  bus_selector : BusSelector  OutputSignals=AirAmbTe_D_Qf,AirAmb_P_Actl,AirAmb_Te_Actl,AirAmb_Te_ActlFilt,AslChime_B_Rq,AslIconDsply_D_Rq,DynoMde_B_Cmd,EcssLamp_D_RqDsply,EngAout_Aa_Actl,GasPrtc_D_RqDsply,HvacHtrCore2_Te_Actl
  wires:
  in_port/1 -> bus_selector/1  "EngineClimateData_Ox178"
  bus_selector/1 -> AirAmbTe_D_Qf/1  "<AirAmbTe_D_Qf>"
  bus_selector/2 -> AirAmb_P_Actl/1  "<AirAmb_P_Actl>"
  bus_selector/3 -> AirAmb_Te_Actl/1  "<AirAmb_Te_Actl>"
  bus_selector/4 -> AirAmb_Te_ActlFilt/1  "<AirAmb_Te_ActlFilt>"
  bus_selector/5 -> AslChime_B_Rq/1  "<AslChime_B_Rq>"
  bus_selector/6 -> AslIconDsply_D_Rq/1  "<AslIconDsply_D_Rq>"
  bus_selector/7 -> DynoMde_B_Cmd/1  "<DynoMde_B_Cmd>"
  bus_selector/8 -> EcssLamp_D_RqDsply/1  "<EcssLamp_D_RqDsply>"
  bus_selector/9 -> EngAout_Aa_Actl/1  "<EngAout_Aa_Actl>"
  bus_selector/10 -> GasPrtc_D_RqDsply/1  "<GasPrtc_D_RqDsply>"
  bus_selector/11 -> HvacHtrCore2_Te_Actl/1  "<HvacHtrCore2_Te_Actl>"

== system test_mdl_NI/Subsystem/ECM_Diesel/EngineData_10_Ox163 ==
  in_port : Inport
  AccFllwMdeActv_B_Actl : Terminator
  AutoRgenTxt_B_RqDsply : Terminator
  DieslMsgTxt_D_Rq : Terminator
  EngPtoMde_D_Actl : Terminator
  ManRgenSoot_Pc_RqDsply : Terminator
  ManRgenTxt_D_RqDsply : Terminator
  bus_selector : BusSelector  OutputSignals=AccFllwMdeActv_B_Actl,AutoRgenTxt_B_RqDsply,DieslMsgTxt_D_Rq,EngPtoMde_D_Actl,ManRgenSoot_Pc_RqDsply,ManRgenTxt_D_RqDsply
  wires:
  in_port/1 -> bus_selector/1  "EngineData_10_Ox163"
  bus_selector/1 -> AccFllwMdeActv_B_Actl/1  "<AccFllwMdeActv_B_Actl>"
  bus_selector/2 -> AutoRgenTxt_B_RqDsply/1  "<AutoRgenTxt_B_RqDsply>"
  bus_selector/3 -> DieslMsgTxt_D_Rq/1  "<DieslMsgTxt_D_Rq>"
  bus_selector/4 -> EngPtoMde_D_Actl/1  "<EngPtoMde_D_Actl>"
  bus_selector/5 -> ManRgenSoot_Pc_RqDsply/1  "<ManRgenSoot_Pc_RqDsply>"
  bus_selector/6 -> ManRgenTxt_D_RqDsply/1  "<ManRgenTxt_D_RqDsply>"

== system test_mdl_NI/Subsystem/ECM_Diesel/EngineData_11_Ox175 ==
  in_port : Inport
  DieslPrtc2_D_RqDsply : Terminator
  DieslPrtcRgen_D_Actl : Terminator
  EngExhOvrTe_B_RqDsply : Terminator
  EngTeColdPrtct_D_Stats : Terminator
  bus_selector : BusSelector  OutputSignals=DieslPrtc2_D_RqDsply,DieslPrtcRgen_D_Actl,EngExhOvrTe_B_RqDsply,EngTeColdPrtct_D_Stats
  wires:
  in_port/1 -> bus_selector/1  "EngineData_11_Ox175"
  bus_selector/1 -> DieslPrtc2_D_RqDsply/1  "<DieslPrtc2_D_RqDsply>"
  bus_selector/2 -> DieslPrtcRgen_D_Actl/1  "<DieslPrtcRgen_D_Actl>"
  bus_selector/3 -> EngExhOvrTe_B_RqDsply/1  "<EngExhOvrTe_B_RqDsply>"
  bus_selector/4 -> EngTeColdPrtct_D_Stats/1  "<EngTeColdPrtct_D_Stats>"

== system test_mdl_NI/Subsystem/ECM_Diesel/EngineData_16_Ox17C ==
  in_port : Inport
  EngAout_N_MxAllw : Terminator
  EngExhBrkAutoLamp_B_Rq : Terminator
  EngExhBrkMde_D_Actl : Terminator
  EngExhBrkOnLamp_B_Rq : Terminator
  EngOilLvlWarn_D_Rq1 : Terminator
  bus_selector : BusSelector  OutputSignals=EngAout_N_MxAllw,EngExhBrkAutoLamp_B_Rq,EngExhBrkMde_D_Actl,EngExhBrkOnLamp_B_Rq,EngOilLvlWarn_D_Rq1
  wires:
  in_port/1 -> bus_selector/1  "EngineData_16_Ox17C"
  bus_selector/1 -> EngAout_N_MxAllw/1  "<EngAout_N_MxAllw>"
  bus_selector/2 -> EngExhBrkAutoLamp_B_Rq/1  "<EngExhBrkAutoLamp_B_Rq>"
  bus_selector/3 -> EngExhBrkMde_D_Actl/1  "<EngExhBrkMde_D_Actl>"
  bus_selector/4 -> EngExhBrkOnLamp_B_Rq/1  "<EngExhBrkOnLamp_B_Rq>"
  bus_selector/5 -> EngOilLvlWarn_D_Rq1/1  "<EngOilLvlWarn_D_Rq1>"

== system test_mdl_NI/Subsystem/ECM_Diesel/EngineData_17_Ox17D ==
  in_port : Inport
  DistToNextOilChange : Terminator
  EngOilLife_T_Actl : Terminator
  EngOilSrvcMsgTxt_D_Rq : Terminator
  GlowIndication : Terminator
  RunDryPrevent_B_Stat : Terminator
  WaterInFuel : Terminator
  bus_selector : BusSelector  OutputSignals=DistToNextOilChange,EngOilLife_T_Actl,EngOilSrvcMsgTxt_D_Rq,GlowIndication,RunDryPrevent_B_Stat,WaterInFuel
  wires:
  in_port/1 -> bus_selector/1  "EngineData_17_Ox17D"
  bus_selector/1 -> DistToNextOilChange/1  "<DistToNextOilChange>"
  bus_selector/2 -> EngOilLife_T_Actl/1  "<EngOilLife_T_Actl>"
  bus_selector/3 -> EngOilSrvcMsgTxt_D_Rq/1  "<EngOilSrvcMsgTxt_D_Rq>"
  bus_selector/4 -> GlowIndication/1  "<GlowIndication>"
  bus_selector/5 -> RunDryPrevent_B_Stat/1  "<RunDryPrevent_B_Stat>"
  bus_selector/6 -> WaterInFuel/1  "<WaterInFuel>"

== system test_mdl_NI/Subsystem/ECM_Diesel/EngineData_6_Ox156 ==
  in_port : Inport
  EngClntTe_D_Qf : Terminator
  EngClnt_Te_Actl : Terminator
  EngGoutLss_Tq_Est : Terminator
  EngOil_Te_Actl : Terminator
  EngOvrhtMitgActv_D_Ind : Terminator
  bus_selector : BusSelector  OutputSignals=EngClntTe_D_Qf,EngClnt_Te_Actl,EngGoutLss_Tq_Est,EngOil_Te_Actl,EngOvrhtMitgActv_D_Ind
  wires:
  in_port/1 -> bus_selector/1  "EngineData_6_Ox156"
  bus_selector/1 -> EngClntTe_D_Qf/1  "<EngClntTe_D_Qf>"
  bus_selector/2 -> EngClnt_Te_Actl/1  "<EngClnt_Te_Actl>"
  bus_selector/3 -> EngGoutLss_Tq_Est/1  "<EngGoutLss_Tq_Est>"
  bus_selector/4 -> EngOil_Te_Actl/1  "<EngOil_Te_Actl>"
  bus_selector/5 -> EngOvrhtMitgActv_D_Ind/1  "<EngOvrhtMitgActv_D_Ind>"

== system test_mdl_NI/Subsystem/ECM_Diesel/EngineData_7_Ox179 ==
  in_port : Inport
  AirCondClutch_B_Stats : Terminator
  AirCondRec_B_Rq : Terminator
  EngOilLife_Pc_Actl : Terminator
  EngSrvcRqd_B_Rq : Terminator
  FuelFillInlet_B_Dsply : Terminator
  FuelFilterLamp_B_Dsply : Terminator
  FuelFlw_Vl_Dsply : Terminator
  HvacAirFullOut_B_Rq : Terminator
  OdoCount : Terminator
  bus_selector : BusSelector  OutputSignals=AirCondClutch_B_Stats,AirCondRec_B_Rq,EngOilLife_Pc_Actl,EngSrvcRqd_B_Rq,FuelFillInlet_B_Dsply,FuelFilterLamp_B_Dsply,FuelFlw_Vl_Dsply,HvacAirFullOut_B_Rq,OdoCount
  wires:
  in_port/1 -> bus_selector/1  "EngineData_7_Ox179"
  bus_selector/1 -> AirCondClutch_B_Stats/1  "<AirCondClutch_B_Stats>"
  bus_selector/2 -> AirCondRec_B_Rq/1  "<AirCondRec_B_Rq>"
  bus_selector/3 -> EngOilLife_Pc_Actl/1  "<EngOilLife_Pc_Actl>"
  bus_selector/4 -> EngSrvcRqd_B_Rq/1  "<EngSrvcRqd_B_Rq>"
  bus_selector/5 -> FuelFillInlet_B_Dsply/1  "<FuelFillInlet_B_Dsply>"
  bus_selector/6 -> FuelFilterLamp_B_Dsply/1  "<FuelFilterLamp_B_Dsply>"
  bus_selector/7 -> FuelFlw_Vl_Dsply/1  "<FuelFlw_Vl_Dsply>"
  bus_selector/8 -> HvacAirFullOut_B_Rq/1  "<HvacAirFullOut_B_Rq>"
  bus_selector/9 -> OdoCount/1  "<OdoCount>"

== system test_mdl_NI/Subsystem/ECM_Diesel/Engine_Clutch_Data_Ox42F ==
  in_port : Inport
  CluPdlPosPcMeas_D_Qf : Terminator
  CluPdlPos_Pc_Meas : Terminator
  CluPdl_PcRate_Actl : Terminator
  EngAoutIdl_N_Ntrl : Terminator
  EngAout_N_Dsply : Terminator
  bus_selector : BusSelector  OutputSignals=CluPdlPosPcMeas_D_Qf,CluPdlPos_Pc_Meas,CluPdl_PcRate_Actl,EngAoutIdl_N_Ntrl,EngAout_N_Dsply
  wires:
  in_port/1 -> bus_selector/1  "Engine_Clutch_Data_Ox42F"
  bus_selector/1 -> CluPdlPosPcMeas_D_Qf/1  "<CluPdlPosPcMeas_D_Qf>"
  bus_selector/2 -> CluPdlPos_Pc_Meas/1  "<CluPdlPos_Pc_Meas>"
  bus_selector/3 -> CluPdl_PcRate_Actl/1  "<CluPdl_PcRate_Actl>"
  bus_selector/4 -> EngAoutIdl_N_Ntrl/1  "<EngAoutIdl_N_Ntrl>"
  bus_selector/5 -> EngAout_N_Dsply/1  "<EngAout_N_Dsply>"

== system test_mdl_NI/Subsystem/ECM_Diesel/Engine_Data_18_Ox20B ==
  in_port : Inport
  EngAirFiltMsgTxt_D_Rq : Terminator
  UreaMnAdd_L2_Actl : Terminator
  UreaMxAdd_L2_Actl : Terminator
  VehUreaRnge3_L_DsplyMx : Terminator
  WaterInFuel_B_Falt : Terminator
  bus_selector : BusSelector  OutputSignals=EngAirFiltMsgTxt_D_Rq,UreaMnAdd_L2_Actl,UreaMxAdd_L2_Actl,VehUreaRnge3_L_DsplyMx,WaterInFuel_B_Falt
  wires:
  in_port/1 -> bus_selector/1  "Engine_Data_18_Ox20B"
  bus_selector/1 -> EngAirFiltMsgTxt_D_Rq/1  "<EngAirFiltMsgTxt_D_Rq>"
  bus_selector/2 -> UreaMnAdd_L2_Actl/1  "<UreaMnAdd_L2_Actl>"
  bus_selector/3 -> UreaMxAdd_L2_Actl/1  "<UreaMxAdd_L2_Actl>"
  bus_selector/4 -> VehUreaRnge3_L_DsplyMx/1  "<VehUreaRnge3_L_DsplyMx>"
  bus_selector/5 -> WaterInFuel_B_Falt/1  "<WaterInFuel_B_Falt>"

== system test_mdl_NI/Subsystem/ECM_Diesel/Global_PATS_TargetInfo_Ox47 ==
  in_port : Inport
  bus_selector : BusSelector  OutputSignals=immoTarget1Cmd,immoTarget1Data,immoTarget1Status
  immoTarget1Cmd : Terminator
  immoTarget1Data : Terminator
  immoTarget1Status : Terminator
  wires:
  in_port/1 -> bus_selector/1  "Global_PATS_TargetInfo_Ox47"
  bus_selector/1 -> immoTarget1Cmd/1  "<immoTarget1Cmd>"
  bus_selector/2 -> immoTarget1Data/1  "<immoTarget1Data>"
  bus_selector/3 -> immoTarget1Status/1  "<immoTarget1Status>"

== system test_mdl_NI/Subsystem/ECM_Diesel/Low_Voltage_Power_Data_FD1_Ox43D ==
  in_port : Inport
  PwSrcULoComm_B_Falt : Terminator
  PwSrcULoDcnnt_B_Stat : Terminator
  PwSrcULoFalt_D_Stat : Terminator
  PwSrcULoOvrTe_B_Actl : Terminator
  PwSrcULo_I_Actl : Terminator
  PwSrcULo_I_Mx : Terminator
  PwSrcULo_Pc_Mx : Terminator
  ULoRgenTestMde_B_Stat : Terminator
  bus_selector : BusSelector  OutputSignals=PwSrcULoComm_B_Falt,PwSrcULoDcnnt_B_Stat,PwSrcULoFalt_D_Stat,PwSrcULoOvrTe_B_Actl,PwSrcULo_I_Actl,PwSrcULo_I_Mx,PwSrcULo_Pc_Mx,ULoRgenTestMde_B_Stat
  wires:
  in_port/1 -> bus_selector/1  "Low_Voltage_Power_Data_FD1_Ox43D"
  bus_selector/1 -> PwSrcULoComm_B_Falt/1  "<PwSrcULoComm_B_Falt>"
  bus_selector/2 -> PwSrcULoDcnnt_B_Stat/1  "<PwSrcULoDcnnt_B_Stat>"
  bus_selector/3 -> PwSrcULoFalt_D_Stat/1  "<PwSrcULoFalt_D_Stat>"
  bus_selector/4 -> PwSrcULoOvrTe_B_Actl/1  "<PwSrcULoOvrTe_B_Actl>"
  bus_selector/5 -> PwSrcULo_I_Actl/1  "<PwSrcULo_I_Actl>"
  bus_selector/6 -> PwSrcULo_I_Mx/1  "<PwSrcULo_I_Mx>"
  bus_selector/7 -> PwSrcULo_Pc_Mx/1  "<PwSrcULo_Pc_Mx>"
  bus_selector/8 -> ULoRgenTestMde_B_Stat/1  "<ULoRgenTestMde_B_Stat>"

== system test_mdl_NI/Subsystem/ECM_Diesel/OTAPhysPCMtoGWM_ECG_Ox1B936010 ==
  in_port : Inport
  OTAPhysPCMtoGWM_ECG : Terminator
  bus_selector : BusSelector  OutputSignals=OTAPhysPCMtoGWM_ECG
  wires:
  in_port/1 -> bus_selector/1  "OTAPhysPCMtoGWM_ECG_Ox1B936010"
  bus_selector/1 -> OTAPhysPCMtoGWM_ECG/1  "<OTAPhysPCMtoGWM_ECG>"

== system test_mdl_NI/Subsystem/ECM_Diesel/PARSEDPhysPCMtoGWM_ECG_Ox1BA36010 ==
  in_port : Inport
  PARSEDPhysPCMtoGWM_ECG : Terminator
  bus_selector : BusSelector  OutputSignals=PARSEDPhysPCMtoGWM_ECG
  wires:
  in_port/1 -> bus_selector/1  "PARSEDPhysPCMtoGWM_ECG_Ox1BA36010"
  bus_selector/1 -> PARSEDPhysPCMtoGWM_ECG/1  "<PARSEDPhysPCMtoGWM_ECG>"

== system test_mdl_NI/Subsystem/ECM_Diesel/PARSEDPushPCMtoGWM_ECG_Ox1BB36010 ==
  in_port : Inport
  PARSEDPushPCMtoGWM_ECG : Terminator
  bus_selector : BusSelector  OutputSignals=PARSEDPushPCMtoGWM_ECG
  wires:
  in_port/1 -> bus_selector/1  "PARSEDPushPCMtoGWM_ECG_Ox1BB36010"
  bus_selector/1 -> PARSEDPushPCMtoGWM_ECG/1  "<PARSEDPushPCMtoGWM_ECG>"

== system test_mdl_NI/Subsystem/ECM_Diesel/PCM_AutoSar_NetworkMgmt_Ox595 ==
  in_port : Inport
  PCM_AutoSarNMControl : Terminator
  PCM_AutoSarNMNodeId : Terminator
  PCM_AutoSarNMReserved{1..4} (4 alike) : Terminator
  PCM_GWNMProxy : Terminator
  PCM_GWOnBoardTester : Terminator
  bus_selector : BusSelector  OutputSignals=PCM_AutoSarNMControl,PCM_AutoSarNMNodeId,PCM_AutoSarNMReserved1,PCM_AutoSarNMReserved2,PCM_AutoSarNMReserved3,PCM_AutoSarNMReserved4,PCM_GWNMProxy,PCM_GWOnBoardTester
  wires:
  in_port/1 -> bus_selector/1  "PCM_AutoSar_NetworkMgmt_Ox595"
  bus_selector/1 -> PCM_AutoSarNMControl/1  "<PCM_AutoSarNMControl>"
  bus_selector/2 -> PCM_AutoSarNMNodeId/1  "<PCM_AutoSarNMNodeId>"
  bus_selector/3 -> PCM_AutoSarNMReserved1/1  "<PCM_AutoSarNMReserved1>"
  bus_selector/4 -> PCM_AutoSarNMReserved2/1  "<PCM_AutoSarNMReserved2>"
  bus_selector/5 -> PCM_AutoSarNMReserved3/1  "<PCM_AutoSarNMReserved3>"
  bus_selector/6 -> PCM_AutoSarNMReserved4/1  "<PCM_AutoSarNMReserved4>"
  bus_selector/7 -> PCM_GWNMProxy/1  "<PCM_GWNMProxy>"
  bus_selector/8 -> PCM_GWOnBoardTester/1  "<PCM_GWOnBoardTester>"

== system test_mdl_NI/Subsystem/ECM_Diesel/PCM_Rapid_Data_Response_1_Ox6A0 ==
  in_port : Inport
  UUDTPCMResponse1 : Terminator
  bus_selector : BusSelector  OutputSignals=UUDTPCMResponse1
  wires:
  in_port/1 -> bus_selector/1  "PCM_Rapid_Data_Response_1_Ox6A0"
  bus_selector/1 -> UUDTPCMResponse1/1  "<UUDTPCMResponse1>"

== system test_mdl_NI/Subsystem/ECM_Diesel/PCM_Rapid_Data_Response_2_Ox6A1 ==
  in_port : Inport
  UUDTPCMResponse2 : Terminator
  bus_selector : BusSelector  OutputSignals=UUDTPCMResponse2
  wires:
  in_port/1 -> bus_selector/1  "PCM_Rapid_Data_Response_2_Ox6A1"
  bus_selector/1 -> UUDTPCMResponse2/1  "<UUDTPCMResponse2>"

== system test_mdl_NI/Subsystem/ECM_Diesel/PowertrainData_11_Ox232 ==
  in_port : Inport
  GearNtrl_D_Stat : Terminator
  GearNtrl_No_Cnt : Terminator
  GearNtrl_No_Cs : Terminator
  bus_selector : BusSelector  OutputSignals=GearNtrl_D_Stat,GearNtrl_No_Cnt,GearNtrl_No_Cs
  wires:
  in_port/1 -> bus_selector/1  "PowertrainData_11_Ox232"
  bus_selector/1 -> GearNtrl_D_Stat/1  "<GearNtrl_D_Stat>"
  bus_selector/2 -> GearNtrl_No_Cnt/1  "<GearNtrl_No_Cnt>"
  bus_selector/3 -> GearNtrl_No_Cs/1  "<GearNtrl_No_Cs>"

== system test_mdl_NI/Subsystem/ECM_Diesel/PowertrainData_12_Ox203 ==
  in_port : Inport
  PtIgnSwtch_D_Stat : Terminator
  PtIgnSwtch_No_Cnt : Terminator
  PtIgnSwtch_No_Cs : Terminator
  bus_selector : BusSelector  OutputSignals=PtIgnSwtch_D_Stat,PtIgnSwtch_No_Cnt,PtIgnSwtch_No_Cs
  wires:
  in_port/1 -> bus_selector/1  "PowertrainData_12_Ox203"
  bus_selector/1 -> PtIgnSwtch_D_Stat/1  "<PtIgnSwtch_D_Stat>"
  bus_selector/2 -> PtIgnSwtch_No_Cnt/1  "<PtIgnSwtch_No_Cnt>"
  bus_selector/3 -> PtIgnSwtch_No_Cs/1  "<PtIgnSwtch_No_Cs>"

== system test_mdl_NI/Subsystem/ECM_Diesel/PowertrainData_1_Ox421 ==
  in_port : Inport
  AirCondFluidHi_P_Actl : Terminator
  CoolantFanStepAct : Terminator
  ECMMILRequest : Terminator
  EngIdlShutDown_D_Stat : Terminator
  EngIdlShutDwnTxt_D_Rq : Terminator
  FUEL_ALCOHOL_PERCNT : Terminator
  FohEng_D_Rq : Terminator
  OilPressureWarning : Terminator
  TrnTotLss_Tq_Est : Terminator
  TrnTotTq_Rt_Est : Terminator
  VehVLimActv_B_Actl : Terminator
  VehVLimStat_D_Actl : Terminator
  bus_selector : BusSelector  OutputSignals=AirCondFluidHi_P_Actl,CoolantFanStepAct,ECMMILRequest,EngIdlShutDown_D_Stat,EngIdlShutDwnTxt_D_Rq,FUEL_ALCOHOL_PERCNT,FohEng_D_Rq,OilPressureWarning,TrnTotLss_Tq_Est,TrnTotTq_Rt_Est,VehVLimActv_B_Actl,VehVLimStat_D_Actl
  wires:
  in_port/1 -> bus_selector/1  "PowertrainData_1_Ox421"
  bus_selector/1 -> AirCondFluidHi_P_Actl/1  "<AirCondFluidHi_P_Actl>"
  bus_selector/2 -> CoolantFanStepAct/1  "<CoolantFanStepAct>"
  bus_selector/3 -> ECMMILRequest/1  "<ECMMILRequest>"
  bus_selector/4 -> EngIdlShutDown_D_Stat/1  "<EngIdlShutDown_D_Stat>"
  bus_selector/5 -> EngIdlShutDwnTxt_D_Rq/1  "<EngIdlShutDwnTxt_D_Rq>"
  bus_selector/6 -> FUEL_ALCOHOL_PERCNT/1  "<FUEL_ALCOHOL_PERCNT>"
  bus_selector/7 -> FohEng_D_Rq/1  "<FohEng_D_Rq>"
  bus_selector/8 -> OilPressureWarning/1  "<OilPressureWarning>"
  bus_selector/9 -> TrnTotLss_Tq_Est/1  "<TrnTotLss_Tq_Est>"
  bus_selector/10 -> TrnTotTq_Rt_Est/1  "<TrnTotTq_Rt_Est>"
  bus_selector/11 -> VehVLimActv_B_Actl/1  "<VehVLimActv_B_Actl>"
  bus_selector/12 -> VehVLimStat_D_Actl/1  "<VehVLimStat_D_Actl>"

== system test_mdl_NI/Subsystem/ECM_Diesel/PowertrainData_2_Ox42D ==
  in_port : Inport
  ApedPos_Pc_ActlDiag : Terminator
  EngAirIn_Te_Actl : Terminator
  EngClnt_Te_ActlDiag : Terminator
  EngLoad_Pc_CalcDiag : Terminator
  EngMsgTxt_D_Rq : Terminator
  GrllShtrPos_B_Falt : Terminator
  GrllShtrPos_D_Cmd : Terminator
  IsaOffst_D_Stat : Terminator
  ObdWarmUp_B_Complt : Terminator
  SlMde_D_RqDsply : Terminator
  SlMde_D_Stat : Terminator
  bus_selector : BusSelector  OutputSignals=ApedPos_Pc_ActlDiag,EngAirIn_Te_Actl,EngClnt_Te_ActlDiag,EngLoad_Pc_CalcDiag,EngMsgTxt_D_Rq,GrllShtrPos_B_Falt,GrllShtrPos_D_Cmd,IsaOffst_D_Stat,ObdWarmUp_B_Complt,SlMde_D_RqDsply,SlMde_D_Stat
  wires:
  in_port/1 -> bus_selector/1  "PowertrainData_2_Ox42D"
  bus_selector/1 -> ApedPos_Pc_ActlDiag/1  "<ApedPos_Pc_ActlDiag>"
  bus_selector/2 -> EngAirIn_Te_Actl/1  "<EngAirIn_Te_Actl>"
  bus_selector/3 -> EngClnt_Te_ActlDiag/1  "<EngClnt_Te_ActlDiag>"
  bus_selector/4 -> EngLoad_Pc_CalcDiag/1  "<EngLoad_Pc_CalcDiag>"
  bus_selector/5 -> EngMsgTxt_D_Rq/1  "<EngMsgTxt_D_Rq>"
  bus_selector/6 -> GrllShtrPos_B_Falt/1  "<GrllShtrPos_B_Falt>"
  bus_selector/7 -> GrllShtrPos_D_Cmd/1  "<GrllShtrPos_D_Cmd>"
  bus_selector/8 -> IsaOffst_D_Stat/1  "<IsaOffst_D_Stat>"
  bus_selector/9 -> ObdWarmUp_B_Complt/1  "<ObdWarmUp_B_Complt>"
  bus_selector/10 -> SlMde_D_RqDsply/1  "<SlMde_D_RqDsply>"
  bus_selector/11 -> SlMde_D_Stat/1  "<SlMde_D_Stat>"

== system test_mdl_NI/Subsystem/ECM_Diesel/PowertrainData_3_Ox43E ==
  in_port : Inport
  BattULoChrg_U_Cmd : Terminator
  ElLoadCtl_D_Rq : Terminator
  EngMnfld_P_Actl : Terminator
  FuelPumpPwr_B_Rq : Terminator
  bus_selector : BusSelector  OutputSignals=BattULoChrg_U_Cmd,ElLoadCtl_D_Rq,EngMnfld_P_Actl,FuelPumpPwr_B_Rq
  wires:
  in_port/1 -> bus_selector/1  "PowertrainData_3_Ox43E"
  bus_selector/1 -> BattULoChrg_U_Cmd/1  "<BattULoChrg_U_Cmd>"
  bus_selector/2 -> ElLoadCtl_D_Rq/1  "<ElLoadCtl_D_Rq>"
  bus_selector/3 -> EngMnfld_P_Actl/1  "<EngMnfld_P_Actl>"
  bus_selector/4 -> FuelPumpPwr_B_Rq/1  "<FuelPumpPwr_B_Rq>"

== system test_mdl_NI/Subsystem/ECM_Diesel/PowertrainData_6_Ox205 ==
  in_port : Inport
  BrkTot_Tq_RqFapLc : Terminator
  FapLc_B_Err : Terminator
  TrnAin_Pc_RqDrv : Terminator
  bus_selector : BusSelector  OutputSignals=BrkTot_Tq_RqFapLc,FapLc_B_Err,TrnAin_Pc_RqDrv
  wires:
  in_port/1 -> bus_selector/1  "PowertrainData_6_Ox205"
  bus_selector/1 -> BrkTot_Tq_RqFapLc/1  "<BrkTot_Tq_RqFapLc>"
  bus_selector/2 -> FapLc_B_Err/1  "<FapLc_B_Err>"
  bus_selector/3 -> TrnAin_Pc_RqDrv/1  "<TrnAin_Pc_RqDrv>"

== system test_mdl_NI/Subsystem/ECM_Diesel/PowertrainData_7_Ox41F ==
  in_port : Inport
  EcoCochA_Pc_Dsply : Terminator
  EcoCochCrus_Pc_Dsply : Terminator
  EcoCochDecel_Pc_Dsply : Terminator
  EcoCochIdlFuel_Pc_Dsply : Terminator
  EcoCochInstNeg_B_Dsply : Terminator
  EcoCochInst_Pc_Dsply : Terminator
  EcoCochShif_Pc_Dsply : Terminator
  bus_selector : BusSelector  OutputSignals=EcoCochA_Pc_Dsply,EcoCochCrus_Pc_Dsply,EcoCochDecel_Pc_Dsply,EcoCochIdlFuel_Pc_Dsply,EcoCochInstNeg_B_Dsply,EcoCochInst_Pc_Dsply,EcoCochShif_Pc_Dsply
  wires:
  in_port/1 -> bus_selector/1  "PowertrainData_7_Ox41F"
  bus_selector/1 -> EcoCochA_Pc_Dsply/1  "<EcoCochA_Pc_Dsply>"
  bus_selector/2 -> EcoCochCrus_Pc_Dsply/1  "<EcoCochCrus_Pc_Dsply>"
  bus_selector/3 -> EcoCochDecel_Pc_Dsply/1  "<EcoCochDecel_Pc_Dsply>"
  bus_selector/4 -> EcoCochIdlFuel_Pc_Dsply/1  "<EcoCochIdlFuel_Pc_Dsply>"
  bus_selector/5 -> EcoCochInstNeg_B_Dsply/1  "<EcoCochInstNeg_B_Dsply>"
  bus_selector/6 -> EcoCochInst_Pc_Dsply/1  "<EcoCochInst_Pc_Dsply>"
  bus_selector/7 -> EcoCochShif_Pc_Dsply/1  "<EcoCochShif_Pc_Dsply>"

== system test_mdl_NI/Subsystem/ECM_Diesel/PowertrainData_9_Ox44C ==
  in_port : Inport
  AutoTowActv_B_Stat : Terminator
  AutoTowAllw_D_StatMnu : Terminator
  EngExhMdeQuiet_D2_Stat : Terminator
  GrossTrainWeight_M_Est : Terminator
  HvacCmprLim_D_Stat : Terminator
  TrailCtlPt_B_Falt : Terminator
  Veh_V_DsplyTrailCtlSet : Terminator
  WakeAlarm1_B_Typ : Terminator
  WakeAlarm1_T_Rq : Terminator
  bus_selector : BusSelector  OutputSignals=AutoTowActv_B_Stat,AutoTowAllw_D_StatMnu,EngExhMdeQuiet_D2_Stat,GrossTrainWeight_M_Est,HvacCmprLim_D_Stat,TrailCtlPt_B_Falt,Veh_V_DsplyTrailCtlSet,WakeAlarm1_B_Typ,WakeAlarm1_T_Rq
  wires:
  in_port/1 -> bus_selector/1  "PowertrainData_9_Ox44C"
  bus_selector/1 -> AutoTowActv_B_Stat/1  "<AutoTowActv_B_Stat>"
  bus_selector/2 -> AutoTowAllw_D_StatMnu/1  "<AutoTowAllw_D_StatMnu>"
  bus_selector/3 -> EngExhMdeQuiet_D2_Stat/1  "<EngExhMdeQuiet_D2_Stat>"
  bus_selector/4 -> GrossTrainWeight_M_Est/1  "<GrossTrainWeight_M_Est>"
  bus_selector/5 -> HvacCmprLim_D_Stat/1  "<HvacCmprLim_D_Stat>"
  bus_selector/6 -> TrailCtlPt_B_Falt/1  "<TrailCtlPt_B_Falt>"
  bus_selector/7 -> Veh_V_DsplyTrailCtlSet/1  "<Veh_V_DsplyTrailCtlSet>"
  bus_selector/8 -> WakeAlarm1_B_Typ/1  "<WakeAlarm1_B_Typ>"
  bus_selector/9 -> WakeAlarm1_T_Rq/1  "<WakeAlarm1_T_Rq>"
